simulink model "Four_DoF_02_2023b"  (R2024a)
settings: Solver=ode1be  StartTime=0.0  StopTime=inf  FixedStep=0.001  RelTol=1e-3
undefined symbols (not defined in the file or in its folder): X, Y, Z
libraries: sm_lib x127, nesl_utility x70, robotcorelib x6
(part 3 of 3)

== system Four_DoF_02_2023b/Gravity Corn(FF controller)1 ==
  note: mgLsin(zeta)
  q : Inport
  Sin : Trigonometry
  mg : Gain  Gain=1*9.80665*1
  Out1 : Outport
  wires:
  Sin/1 -> mg/1
  q/1 -> Sin/1
  mg/1 -> Out1/1

== system Four_DoF_02_2023b/Gravity Corn(FF controller)2 ==
  note: mgLsin(zeta)
  q : Inport
  Sin : Trigonometry
  mg : Gain  Gain=1*9.80665*1
  Out1 : Outport
  wires:
  Sin/1 -> mg/1
  q/1 -> Sin/1
  mg/1 -> Out1/1

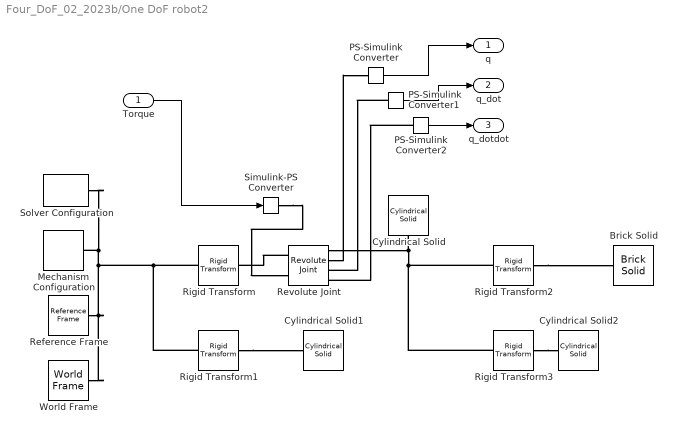
== system Four_DoF_02_2023b/One DoF robot2 ==
  Torque : Inport
  Brick Solid : sm_lib/Body Elements/Brick Solid  BrickDimensions=[0.1 0.1 0.1]  BrickDimensionsUnits=m  ExportEntireGeometry=off  InertiaType=PointMass  BasedOnType=Density  Density=1000  DensityUnits=kg/m^3  Mass=1  MassUnits=kg  CenterOfMass=[0 0 0]  CenterOfMassUnits=m  MomentsOfInertia=[1 1 1]  MomentsOfInertiaUnits=kg*m^2  ProductsOfInertia=[0 0 0]  ProductsOfInertiaUnits=kg*m^2  GraphicType=FromGeometry  MarkerShape=Sphere  MarkerSize=10  GraphicVisPropType=SimpleVisualProperties  GraphicDiffuseColor=[0.5 0.5 0.5]  GraphicOpacity=1.0  GraphicSpecularColor=[0.5 0.5 0.5 1.0]  GraphicAmbientColor=[0.15 0.15 0.15 1.0]  GraphicEmissiveColor=[0.0 0.0 0.0 1.0]  GraphicShininess=75  DoExposeReferenceFrame=on  SerializedFrames=<Frames/>
  Cylindrical Solid : sm_lib/Body Elements/Cylindrical Solid  CylinderRadius=0.05  CylinderRadiusUnits=m  CylinderLength=0.1  CylinderLengthUnits=m  ExportEntireGeometry=off  InertiaType=PointMass  BasedOnType=Density  Density=1000  DensityUnits=kg/m^3  Mass=0.0001  MassUnits=kg  CenterOfMass=[0 0 0]  CenterOfMassUnits=m  MomentsOfInertia=[1 1 1]  MomentsOfInertiaUnits=kg*m^2  ProductsOfInertia=[0 0 0]  ProductsOfInertiaUnits=kg*m^2  GraphicType=FromGeometry  MarkerShape=Sphere  MarkerSize=10  GraphicVisPropType=SimpleVisualProperties  GraphicDiffuseColor=[1.0 0.0 0.2]  GraphicOpacity=1.0  GraphicSpecularColor=[0.5 0.5 0.5 1.0]  GraphicAmbientColor=[0.15 0.15 0.15 1.0]  GraphicEmissiveColor=[0.0 0.0 0.0 1.0]  GraphicShininess=75  DoExposeReferenceFrame=on  SerializedFrames=<Frames/>
  Cylindrical Solid1 : sm_lib/Body Elements/Cylindrical Solid  CylinderRadius=0.02  CylinderRadiusUnits=m  CylinderLength=0.5  CylinderLengthUnits=m  ExportEntireGeometry=off  InertiaType=PointMass  BasedOnType=Density  Density=1000  DensityUnits=kg/m^3  Mass=0.001  MassUnits=kg  CenterOfMass=[0 0 0]  CenterOfMassUnits=m  MomentsOfInertia=[1 1 1]  MomentsOfInertiaUnits=kg*m^2  ProductsOfInertia=[0 0 0]  ProductsOfInertiaUnits=kg*m^2  GraphicType=FromGeometry  MarkerShape=Sphere  MarkerSize=10  GraphicVisPropType=SimpleVisualProperties  GraphicDiffuseColor=[1.0 0.6 0.2]  GraphicOpacity=1.0  GraphicSpecularColor=[0.5 0.5 0.5 1.0]  GraphicAmbientColor=[0.15 0.15 0.15 1.0]  GraphicEmissiveColor=[0.0 0.0 0.0 1.0]  GraphicShininess=75  DoExposeReferenceFrame=on  SerializedFrames=<Frames/>
  Cylindrical Solid2 : sm_lib/Body Elements/Cylindrical Solid  CylinderRadius=0.02  CylinderRadiusUnits=m  CylinderLength=1  CylinderLengthUnits=m  ExportEntireGeometry=off  InertiaType=PointMass  BasedOnType=Density  Density=1000  DensityUnits=kg/m^3  Mass=0.001  MassUnits=kg  CenterOfMass=[0 0 0]  CenterOfMassUnits=m  MomentsOfInertia=[1 1 1]  MomentsOfInertiaUnits=kg*m^2  ProductsOfInertia=[0 0 0]  ProductsOfInertiaUnits=kg*m^2  GraphicType=FromGeometry  MarkerShape=Sphere  MarkerSize=10  GraphicVisPropType=SimpleVisualProperties  GraphicDiffuseColor=[1.0 0.6 0.2]  GraphicOpacity=1.0  GraphicSpecularColor=[0.5 0.5 0.5 1.0]  GraphicAmbientColor=[0.15 0.15 0.15 1.0]  GraphicEmissiveColor=[0.0 0.0 0.0 1.0]  GraphicShininess=75  DoExposeReferenceFrame=on  SerializedFrames=<Frames/>
  Mechanism Configuration : sm_lib/Utilities/Mechanism Configuration  UniformGravity=Constant  GravityVector=[0 0 -9.80665]  GravityVectorUnits=m/s^2  LinearizationDelta=0.001  JointModeTransitionNonlinearIterations=2
  PS-Simulink Converter : nesl_utility/PS-Simulink Converter  PhysicalDomain=network_engine_domain  SubClassName=ps_output  LeftPortType=input  RightPortType=output  PseudoPeriodic=off  Frequencies=[]  VectorFormat=inherit  Unit=inherit  AffineConversion=off
  PS-Simulink Converter1 : nesl_utility/PS-Simulink Converter  PhysicalDomain=network_engine_domain  SubClassName=ps_output  LeftPortType=input  RightPortType=output  PseudoPeriodic=off  Frequencies=[]  VectorFormat=inherit  Unit=inherit  AffineConversion=off
  PS-Simulink Converter2 : nesl_utility/PS-Simulink Converter  PhysicalDomain=network_engine_domain  SubClassName=ps_output  LeftPortType=input  RightPortType=output  PseudoPeriodic=off  Frequencies=[]  VectorFormat=inherit  Unit=inherit  AffineConversion=off
  Reference Frame : sm_lib/Frames and Transforms/Reference Frame
  Revolute Joint : sm_lib/Joints/Revolute Joint  JointMode=Normal  CompositeWrenchDir=FollowerOnBase  CompositeWrenchFrame=BaseFrame  SenseConstraintForce=off  SenseConstraintTorque=off  SenseTotalForce=off  SenseTotalTorque=off  PositionTargetSpecify=on  PositionTargetPriority=High  PositionTargetValue=45  PositionTargetValueUnits=deg  VelocityTargetSpecify=off  VelocityTargetPriority=High  VelocityTargetValue=0  VelocityTargetValueUnits=deg/s  EquilibriumPosition=0  EquilibriumPositionUnits=deg  SpringStiffness=0  SpringStiffnessUnits=N*m/deg  DampingCoefficient=0.01  DampingCoefficientUnits=N*m/(deg/s)  LowerLimitSpecify=off  LowerLimitBound=-90  LowerLimitBoundUnits=deg  LowerLimitStiffness=1e4  LowerLimitStiffnessUnits=N*m/deg  LowerLimitDamping=10  LowerLimitDampingUnits=N*m/(deg/s)  LowerLimitTransitionRegionWidth=0.1  LowerLimitTransitionRegionWidthUnits=deg  UpperLimitSpecify=off  UpperLimitBound=90  UpperLimitBoundUnits=deg  UpperLimitStiffness=1e4  UpperLimitStiffnessUnits=N*m/deg  UpperLimitDamping=10  UpperLimitDampingUnits=N*m/(deg/s)  UpperLimitTransitionRegionWidth=0.1  UpperLimitTransitionRegionWidthUnits=deg  TorqueActuationMode=InputTorque  MotionActuationMode=ComputedMotion  SensePosition=on  SenseVelocity=on  SenseAcceleration=on  SenseTorqueForce=off  SenseLowerLimitTorqueForce=off  SenseUpperLimitTorqueForce=off
  Rigid Transform : sm_lib/Frames and Transforms/Rigid Transform  RotationMethod=StandardAxis  FollAlignAxisA=+X  BaseAlignAxisA=+Y  FollAlignAxisB=+Y  BaseAlignAxisB=+Z  RotationStandardAxis=+Y  RotationAngle=90  RotationAngleUnits=deg  RotationArbitraryAxis=[0 0 1]  RotationSequenceAxes=FollowerAxes  RotationSequence=XYX  RotationSequenceAngles=[0 0 0]  RotationSequenceAnglesUnits=deg  RotationMatrix=[1 0 0; 0 1 0; 0 0 1]  Quaternion=[1 0 0 0]  TranslationMethod=Cartesian  TranslationCartesianOffset=[0 0 0.5]  TranslationCartesianOffsetUnits=m  TranslationStandardAxis=+Z  TranslationStandardOffset=0  TranslationStandardOffsetUnits=m  TranslationROffset=0  TranslationROffsetUnits=m  TranslationThetaOffset=0  TranslationThetaOffsetUnits=deg  TranslationZOffset=0  TranslationZOffsetUnits=m
  Rigid Transform1 : sm_lib/Frames and Transforms/Rigid Transform  RotationMethod=None  FollAlignAxisA=+X  BaseAlignAxisA=+Y  FollAlignAxisB=+Y  BaseAlignAxisB=+Z  RotationStandardAxis=+Y  RotationAngle=90  RotationAngleUnits=deg  RotationArbitraryAxis=[0 0 1]  RotationSequenceAxes=FollowerAxes  RotationSequence=XYX  RotationSequenceAngles=[0 0 0]  RotationSequenceAnglesUnits=deg  RotationMatrix=[1 0 0; 0 1 0; 0 0 1]  Quaternion=[1 0 0 0]  TranslationMethod=Cartesian  TranslationCartesianOffset=[0 0 0.25]  TranslationCartesianOffsetUnits=m  TranslationStandardAxis=+Z  TranslationStandardOffset=0  TranslationStandardOffsetUnits=m  TranslationROffset=0  TranslationROffsetUnits=m  TranslationThetaOffset=0  TranslationThetaOffsetUnits=deg  TranslationZOffset=0  TranslationZOffsetUnits=m
  Rigid Transform2 : sm_lib/Frames and Transforms/Rigid Transform  RotationMethod=None  FollAlignAxisA=+X  BaseAlignAxisA=+Y  FollAlignAxisB=+Y  BaseAlignAxisB=+Z  RotationStandardAxis=+Z  RotationAngle=0.0  RotationAngleUnits=deg  RotationArbitraryAxis=[0 0 1]  RotationSequenceAxes=FollowerAxes  RotationSequence=XYX  RotationSequenceAngles=[0 0 0]  RotationSequenceAnglesUnits=deg  RotationMatrix=[1 0 0; 0 1 0; 0 0 1]  Quaternion=[1 0 0 0]  TranslationMethod=Cartesian  TranslationCartesianOffset=[1 0 0]  TranslationCartesianOffsetUnits=m  TranslationStandardAxis=+Z  TranslationStandardOffset=0  TranslationStandardOffsetUnits=m  TranslationROffset=0  TranslationROffsetUnits=m  TranslationThetaOffset=0  TranslationThetaOffsetUnits=deg  TranslationZOffset=0  TranslationZOffsetUnits=m
  Rigid Transform3 : sm_lib/Frames and Transforms/Rigid Transform  RotationMethod=StandardAxis  FollAlignAxisA=+X  BaseAlignAxisA=+Y  FollAlignAxisB=+Y  BaseAlignAxisB=+Z  RotationStandardAxis=+Y  RotationAngle=90  RotationAngleUnits=deg  RotationArbitraryAxis=[0 0 1]  RotationSequenceAxes=FollowerAxes  RotationSequence=XYX  RotationSequenceAngles=[0 0 0]  RotationSequenceAnglesUnits=deg  RotationMatrix=[1 0 0; 0 1 0; 0 0 1]  Quaternion=[1 0 0 0]  TranslationMethod=Cartesian  TranslationCartesianOffset=[0.5 0 0]  TranslationCartesianOffsetUnits=m  TranslationStandardAxis=+Z  TranslationStandardOffset=0  TranslationStandardOffsetUnits=m  TranslationROffset=0  TranslationROffsetUnits=m  TranslationThetaOffset=0  TranslationThetaOffsetUnits=deg  TranslationZOffset=0  TranslationZOffsetUnits=m
  Simulink-PS Converter : nesl_utility/Simulink-PS Converter  PhysicalDomain=network_engine_domain  SubClassName=ps_input  LeftPortType=input  RightPortType=output  PseudoPeriodic=off  Frequencies=[]  NoiseDistribution=none  NoiseParameters=[]  Unit=1  AffineConversion=off  FilteringAndDerivatives=provide  SimscapeFilterOrder=1  InputFilterTimeConstant=0.001  UdotUserProvided=0
  Solver Configuration : nesl_utility/Solver Configuration  PhysicalDomain=network_engine_domain  SubClassName=solver  LeftPortType=input  RightPortType=generic  Tones=[]  Harmonics=[]  SimulateNoise=off  Profile=off  UseLocalSampling=off  EnableSwitchedLinearOptims=on  FrequencyDomain=off  UseCCode=off  RelTol=0.001  AbsTol=0.001  MinStep=1e-09  ToWorkspace=off  RevertToSquareIcSolve=off  NumHomotopyIterations=100  PhasorMode=off  PhasorModeNumHarmonics=1  ConsistencySolver=NEWTON_XTOL_AFTER_FTOL  IndexReductionMethod=DerivativeReplacement  DoDC=off  ResidualTolerance=1e-09  ConsistencyTolSource=GLOBAL  ConsistencyAbsTol=0.001  ConsistencyRelTol=0.001  ConsistencyTolFactor=0.001  UseLocalSolver=off  LocalSolverChoice=NE_BACKWARD_EULER_ADVANCER  ResolveIndetEquations=on  FunctionEvalNumThread=1  LocalSolverSampleTime=0.001  DoFixedCost=off  MaxNonlinIter=3  MaxModeIter=2  ComputeImpulses=off  ImpulseIterations=2  LinearAlgebra=auto  LinearAlgebraNumThread=0  EquationFormulation=NE_TIME_EF  DelaysMemoryBudget=1024  AutomaticFiltering=on  FilteringTimeConstant=0.001  PartitionStorageMethod=AS_NEEDED  PartitionMemoryBudget=1024  PartitionMethod=ROBUST  MultibodyUseLocalSolver=off  MultibodyLocalSolverChoice=ODE1  MultibodyLocalSolverSampleTime=0.001
  World Frame : sm_lib/Frames and Transforms/World Frame
  q : Outport
  q_dot : Outport  Port=2
  q_dotdot : Outport  Port=3
  wires:
  Torque/1 -> Simulink-PS Converter/1
  PS-Simulink Converter/1 -> q/1
  PS-Simulink Converter2/1 -> q_dotdot/1
  PS-Simulink Converter1/1 -> q_dot/1
  connections:
  Solver Configuration/RConn1 -- Rigid Transform1/LConn1 -- Rigid Transform/LConn1 -- World Frame/RConn1 -- Reference Frame/RConn1 -- Mechanism Configuration/RConn1
  Revolute Joint/RConn1 -- Rigid Transform3/LConn1 -- Rigid Transform2/LConn1 -- Cylindrical Solid/RConn1
  Revolute Joint/LConn1 -- Rigid Transform/RConn1
  Rigid Transform3/RConn1 -- Cylindrical Solid2/RConn1
  Rigid Transform1/RConn1 -- Cylindrical Solid1/RConn1
  PS-Simulink Converter2/LConn1 -- Revolute Joint/RConn4
  Revolute Joint/RConn2 -- PS-Simulink Converter/LConn1
  Rigid Transform2/RConn1 -- Brick Solid/RConn1
  Simulink-PS Converter/RConn1 -- Revolute Joint/LConn2
  PS-Simulink Converter1/LConn1 -- Revolute Joint/RConn3

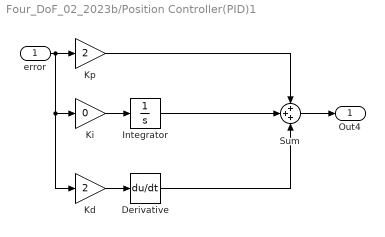
== system Four_DoF_02_2023b/Position Controller(PID)1 ==
  error : Inport
  Derivative : Derivative
  Integrator : Integrator
  Kd : Gain  Gain=2
  Ki : Gain  Gain=0
  Kp : Gain  Gain=2
  Sum : Sum  Inputs=+++
  Out4 : Outport
  wires:
  Derivative/1 -> Sum/3
  Ki/1 -> Integrator/1
  Integrator/1 -> Sum/2
  Kd/1 -> Derivative/1
  Kp/1 -> Sum/1
  error/1 -> Kd/1, Ki/1, Kp/1
  Sum/1 -> Out4/1

== system Four_DoF_02_2023b/Position Controller(PID)2 ==
  error : Inport
  Derivative : Derivative
  Integrator : Integrator
  Kd : Gain  Gain=2
  Ki : Gain  Gain=0
  Kp : Gain  Gain=2
  Sum : Sum  Inputs=+++
  Out4 : Outport
  wires:
  Derivative/1 -> Sum/3
  Ki/1 -> Integrator/1
  Integrator/1 -> Sum/2
  Kd/1 -> Derivative/1
  Kp/1 -> Sum/1
  error/1 -> Kd/1, Ki/1, Kp/1
  Sum/1 -> Out4/1

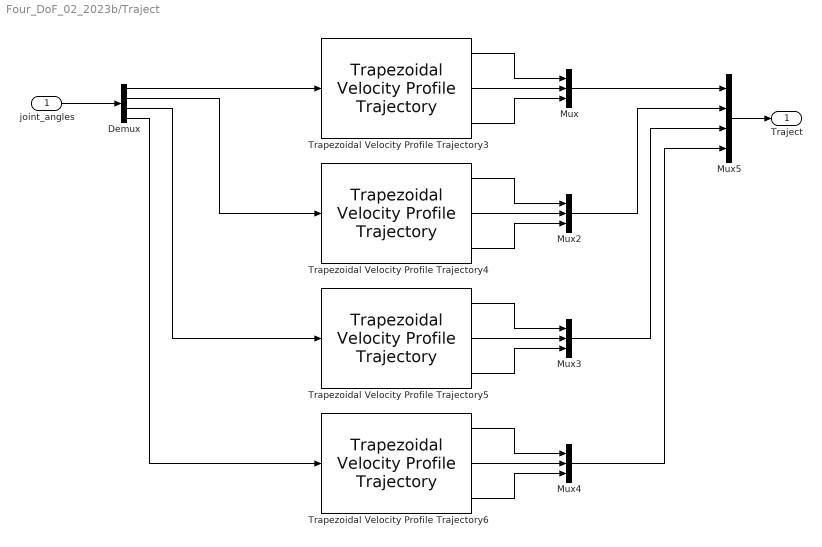
== system Four_DoF_02_2023b/Traject ==
  joint_angles : Inport
  Demux : Demux
  Mux{,2..4} (4 alike) : Mux  Inputs=3
  Mux5 : Mux
  Trapezoidal Velocity Profile Trajectory3 : robotcorelib/Trapezoidal Velocity Profile Trajectory  WaypointSource=Internal  Waypoints=[ 0, 0, 0]  NumParams=0  Parameter1=Peak Velocity  Parameter2=End Time  ParameterSource=Internal  PeakVelocity=[ 2; 2 ]  Acceleration=[ 1; 2 ]  EndTime=[ 1; 1 ]  AccelTime=[ 1; 2 ]  SimulateUsing=Interpreted execution
  Trapezoidal Velocity Profile Trajectory4 : robotcorelib/Trapezoidal Velocity Profile Trajectory  WaypointSource=Internal  Waypoints=[ 0, 0, 0]  NumParams=0  Parameter1=Peak Velocity  Parameter2=End Time  ParameterSource=Internal  PeakVelocity=[ 2; 2 ]  Acceleration=[ 1; 2 ]  EndTime=[ 1; 1 ]  AccelTime=[ 1; 2 ]  SimulateUsing=Interpreted execution
  Trapezoidal Velocity Profile Trajectory5 : robotcorelib/Trapezoidal Velocity Profile Trajectory  WaypointSource=Internal  Waypoints=[ 0, 1, 5]  NumParams=0  Parameter1=Peak Velocity  Parameter2=End Time  ParameterSource=Internal  PeakVelocity=[ 2; 2 ]  Acceleration=[ 1; 2 ]  EndTime=[ 1; 1 ]  AccelTime=[ 1; 2 ]  SimulateUsing=Interpreted execution
  Trapezoidal Velocity Profile Trajectory6 : robotcorelib/Trapezoidal Velocity Profile Trajectory  WaypointSource=Internal  Waypoints=[ 0, 1, 3]  NumParams=0  Parameter1=Peak Velocity  Parameter2=End Time  ParameterSource=Internal  PeakVelocity=[ 2; 2 ]  Acceleration=[ 1; 2 ]  EndTime=[ 1; 1 ]  AccelTime=[ 1; 2 ]  SimulateUsing=Interpreted execution
  Traject : Outport
  wires:
  Trapezoidal Velocity Profile Trajectory5/2 -> Mux3/2
  Mux4/1 -> Mux5/4
  Mux3/1 -> Mux5/3
  Trapezoidal Velocity Profile Trajectory3/2 -> Mux/2
  Trapezoidal Velocity Profile Trajectory6/1 -> Mux4/1
  Mux2/1 -> Mux5/2
  Trapezoidal Velocity Profile Trajectory6/2 -> Mux4/2
  Trapezoidal Velocity Profile Trajectory3/3 -> Mux/3
  Trapezoidal Velocity Profile Trajectory6/3 -> Mux4/3
  Trapezoidal Velocity Profile Trajectory5/3 -> Mux3/3
  Trapezoidal Velocity Profile Trajectory3/1 -> Mux/1
  Mux/1 -> Mux5/1
  Trapezoidal Velocity Profile Trajectory4/3 -> Mux2/3
  Trapezoidal Velocity Profile Trajectory4/1 -> Mux2/1
  Trapezoidal Velocity Profile Trajectory4/2 -> Mux2/2
  Trapezoidal Velocity Profile Trajectory5/1 -> Mux3/1
  Mux5/1 -> Traject/1
  joint_angles/1 -> Demux/1
  Demux/1 -> Trapezoidal Velocity Profile Trajectory3/1
  Demux/2 -> Trapezoidal Velocity Profile Trajectory4/1
  Demux/3 -> Trapezoidal Velocity Profile Trajectory5/1
  Demux/4 -> Trapezoidal Velocity Profile Trajectory6/1

== system Four_DoF_02_2023b/Velocity Controller(PID)1 ==
  error : Inport
  Derivative : Derivative
  Integrator : Integrator
  Kd : Gain  Gain=0
  Ki : Gain  Gain=0
  Kp : Gain  Gain=4
  Sum : Sum  Inputs=+++
  Out4 : Outport
  wires:
  Derivative/1 -> Sum/3
  Ki/1 -> Integrator/1
  Integrator/1 -> Sum/2
  Kd/1 -> Derivative/1
  Kp/1 -> Sum/1
  error/1 -> Kd/1, Ki/1, Kp/1
  Sum/1 -> Out4/1

== system Four_DoF_02_2023b/Velocity Controller(PID)2 ==
  error : Inport
  Derivative : Derivative
  Integrator : Integrator
  Kd : Gain  Gain=0
  Ki : Gain  Gain=0
  Kp : Gain
  Sum : Sum  Inputs=+++
  Torque 2 : Outport
  wires:
  Derivative/1 -> Sum/3
  Ki/1 -> Integrator/1
  Integrator/1 -> Sum/2
  Kd/1 -> Derivative/1
  Kp/1 -> Sum/1
  error/1 -> Kd/1, Ki/1, Kp/1
  Sum/1 -> Torque 2/1

== system Four_DoF_02_2023b/Velocity Controller(PID)3 ==
  error : Inport
  Derivative : Derivative
  Integrator : Integrator
  Kd : Gain  Gain=0
  Ki : Gain  Gain=0
  Kp : Gain  Gain=4
  Sum : Sum  Inputs=+++
  Out4 : Outport
  wires:
  Derivative/1 -> Sum/3
  Ki/1 -> Integrator/1
  Integrator/1 -> Sum/2
  Kd/1 -> Derivative/1
  Kp/1 -> Sum/1
  error/1 -> Kd/1, Ki/1, Kp/1
  Sum/1 -> Out4/1

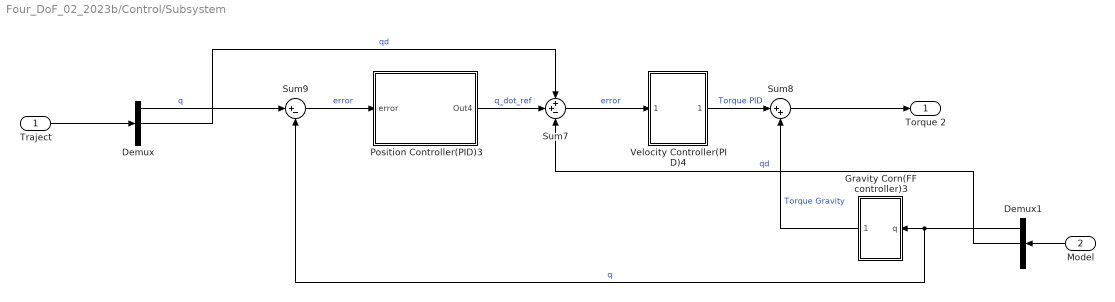
== system Four_DoF_02_2023b/Control/Subsystem ==
  Traject : Inport
  Model : Inport  Port=2
  Demux : Demux  Outputs=3
  Demux1 : Demux  Outputs=3
  Gravity Corn(FF controller)3 : Subsystem
  Position Controller(PID)3 : Subsystem
  Sum7 : Sum  Inputs=++-
  Sum8 : Sum  Inputs=|++
  Sum9 : Sum  Inputs=|+-
  Velocity Controller(PID)4 : Subsystem
  Torque 2 : Outport
  wires:
  Position Controller(PID)3/1(Out4) -> Sum7/2  "q_dot_ref"
  Gravity Corn(FF controller)3/1(Out1) -> Sum8/2  "Torque Gravity"
  Traject/1 -> Demux/1
  Velocity Controller(PID)4/1(Out4) -> Sum8/1  "Torque PID"
  Sum7/1 -> Velocity Controller(PID)4/1(error)  "error"
  Sum9/1 -> Position Controller(PID)3/1(error)  "error"
  Sum8/1 -> Torque 2/1
  Demux/1 -> Sum9/1  "q"
  Demux/2 -> Sum7/1  "qd"
  Model/1 -> Demux1/1
  Demux1/1 -> Sum9/2, Gravity Corn(FF controller)3/1(q)  "q"
  Demux1/2 -> Sum7/3  "qd"

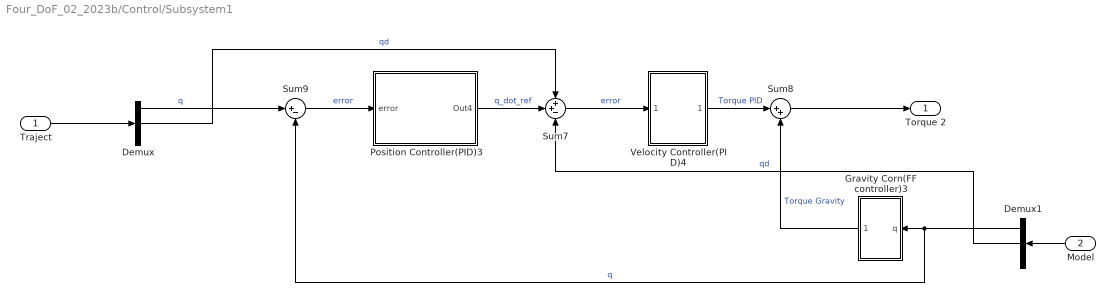
== system Four_DoF_02_2023b/Control/Subsystem1 ==
  Traject : Inport
  Model : Inport  Port=2
  Demux : Demux  Outputs=3
  Demux1 : Demux  Outputs=3
  Gravity Corn(FF controller)3 : Subsystem
  Position Controller(PID)3 : Subsystem
  Sum7 : Sum  Inputs=++-
  Sum8 : Sum  Inputs=|++
  Sum9 : Sum  Inputs=|+-
  Velocity Controller(PID)4 : Subsystem
  Torque 2 : Outport
  wires:
  Position Controller(PID)3/1(Out4) -> Sum7/2  "q_dot_ref"
  Gravity Corn(FF controller)3/1(Out1) -> Sum8/2  "Torque Gravity"
  Traject/1 -> Demux/1
  Velocity Controller(PID)4/1(Out4) -> Sum8/1  "Torque PID"
  Sum7/1 -> Velocity Controller(PID)4/1(error)  "error"
  Sum9/1 -> Position Controller(PID)3/1(error)  "error"
  Sum8/1 -> Torque 2/1
  Demux/1 -> Sum9/1  "q"
  Demux/2 -> Sum7/1  "qd"
  Model/1 -> Demux1/1
  Demux1/1 -> Sum9/2, Gravity Corn(FF controller)3/1(q)  "q"
  Demux1/2 -> Sum7/3  "qd"

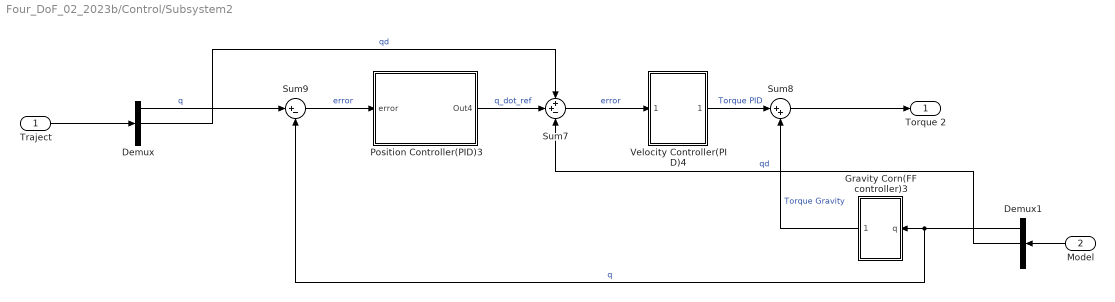
== system Four_DoF_02_2023b/Control/Subsystem2 ==
  Traject : Inport
  Model : Inport  Port=2
  Demux : Demux  Outputs=3
  Demux1 : Demux  Outputs=3
  Gravity Corn(FF controller)3 : Subsystem
  Position Controller(PID)3 : Subsystem
  Sum7 : Sum  Inputs=++-
  Sum8 : Sum  Inputs=|++
  Sum9 : Sum  Inputs=|+-
  Velocity Controller(PID)4 : Subsystem
  Torque 2 : Outport
  wires:
  Position Controller(PID)3/1(Out4) -> Sum7/2  "q_dot_ref"
  Gravity Corn(FF controller)3/1(Out1) -> Sum8/2  "Torque Gravity"
  Traject/1 -> Demux/1
  Velocity Controller(PID)4/1(Out4) -> Sum8/1  "Torque PID"
  Sum7/1 -> Velocity Controller(PID)4/1(error)  "error"
  Sum9/1 -> Position Controller(PID)3/1(error)  "error"
  Sum8/1 -> Torque 2/1
  Demux/1 -> Sum9/1  "q"
  Demux/2 -> Sum7/1  "qd"
  Model/1 -> Demux1/1
  Demux1/1 -> Sum9/2, Gravity Corn(FF controller)3/1(q)  "q"
  Demux1/2 -> Sum7/3  "qd"

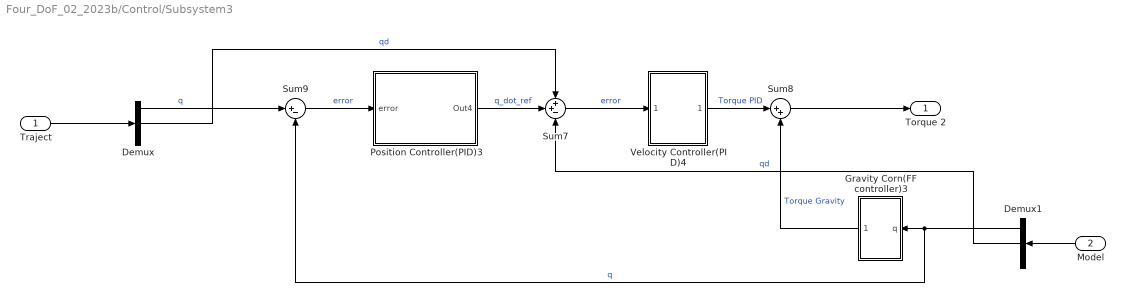
== system Four_DoF_02_2023b/Control/Subsystem3 ==
  Traject : Inport
  Model : Inport  Port=2
  Demux : Demux  Outputs=3
  Demux1 : Demux  Outputs=3
  Gravity Corn(FF controller)3 : Subsystem
  Position Controller(PID)3 : Subsystem
  Sum7 : Sum  Inputs=++-
  Sum8 : Sum  Inputs=|++
  Sum9 : Sum  Inputs=|+-
  Velocity Controller(PID)4 : Subsystem
  Torque 2 : Outport
  wires:
  Position Controller(PID)3/1(Out4) -> Sum7/2  "q_dot_ref"
  Gravity Corn(FF controller)3/1(Out1) -> Sum8/2  "Torque Gravity"
  Traject/1 -> Demux/1
  Velocity Controller(PID)4/1(Out4) -> Sum8/1  "Torque PID"
  Sum7/1 -> Velocity Controller(PID)4/1(error)  "error"
  Sum9/1 -> Position Controller(PID)3/1(error)  "error"
  Sum8/1 -> Torque 2/1
  Demux/1 -> Sum9/1  "q"
  Demux/2 -> Sum7/1  "qd"
  Model/1 -> Demux1/1
  Demux1/1 -> Sum9/2, Gravity Corn(FF controller)3/1(q)  "q"
  Demux1/2 -> Sum7/3  "qd"

== system Four_DoF_02_2023b/Control/Subsystem/Gravity Corn(FF controller)3 ==
  note: mgLsin(zeta)
  q : Inport
  Sin : Trigonometry
  mg : Gain  Gain=1*9.80665*1
  Out1 : Outport
  wires:
  Sin/1 -> mg/1
  q/1 -> Sin/1
  mg/1 -> Out1/1

== system Four_DoF_02_2023b/Control/Subsystem/Position Controller(PID)3 ==
  error : Inport
  Derivative : Derivative
  Integrator : Integrator
  Kd : Gain  Gain=2
  Ki : Gain  Gain=0
  Kp : Gain  Gain=2
  Sum : Sum  Inputs=+++
  Out4 : Outport
  wires:
  Derivative/1 -> Sum/3
  Ki/1 -> Integrator/1
  Integrator/1 -> Sum/2
  Kd/1 -> Derivative/1
  Kp/1 -> Sum/1
  error/1 -> Kd/1, Ki/1, Kp/1
  Sum/1 -> Out4/1

== system Four_DoF_02_2023b/Control/Subsystem/Velocity Controller(PID)4 ==
  error : Inport
  Derivative : Derivative
  Integrator : Integrator
  Kd : Gain  Gain=0
  Ki : Gain  Gain=0
  Kp : Gain  Gain=4
  Sum : Sum  Inputs=+++
  Out4 : Outport
  wires:
  Derivative/1 -> Sum/3
  Ki/1 -> Integrator/1
  Integrator/1 -> Sum/2
  Kd/1 -> Derivative/1
  Kp/1 -> Sum/1
  error/1 -> Kd/1, Ki/1, Kp/1
  Sum/1 -> Out4/1

== system Four_DoF_02_2023b/Control/Subsystem1/Gravity Corn(FF controller)3 ==
  note: mgLsin(zeta)
  q : Inport
  Sin : Trigonometry
  mg : Gain  Gain=1*9.80665*1
  Out1 : Outport
  wires:
  Sin/1 -> mg/1
  q/1 -> Sin/1
  mg/1 -> Out1/1

== system Four_DoF_02_2023b/Control/Subsystem1/Position Controller(PID)3 ==
  error : Inport
  Derivative : Derivative
  Integrator : Integrator
  Kd : Gain  Gain=2
  Ki : Gain  Gain=0
  Kp : Gain  Gain=2
  Sum : Sum  Inputs=+++
  Out4 : Outport
  wires:
  Derivative/1 -> Sum/3
  Ki/1 -> Integrator/1
  Integrator/1 -> Sum/2
  Kd/1 -> Derivative/1
  Kp/1 -> Sum/1
  error/1 -> Kd/1, Ki/1, Kp/1
  Sum/1 -> Out4/1

== system Four_DoF_02_2023b/Control/Subsystem1/Velocity Controller(PID)4 ==
  error : Inport
  Derivative : Derivative
  Integrator : Integrator
  Kd : Gain  Gain=0
  Ki : Gain  Gain=0
  Kp : Gain  Gain=4
  Sum : Sum  Inputs=+++
  Out4 : Outport
  wires:
  Derivative/1 -> Sum/3
  Ki/1 -> Integrator/1
  Integrator/1 -> Sum/2
  Kd/1 -> Derivative/1
  Kp/1 -> Sum/1
  error/1 -> Kd/1, Ki/1, Kp/1
  Sum/1 -> Out4/1

== system Four_DoF_02_2023b/Control/Subsystem2/Gravity Corn(FF controller)3 ==
  note: mgLsin(zeta)
  q : Inport
  Sin : Trigonometry
  mg : Gain  Gain=1*9.80665*1
  Out1 : Outport
  wires:
  Sin/1 -> mg/1
  q/1 -> Sin/1
  mg/1 -> Out1/1

== system Four_DoF_02_2023b/Control/Subsystem2/Position Controller(PID)3 ==
  error : Inport
  Derivative : Derivative
  Integrator : Integrator
  Kd : Gain  Gain=2
  Ki : Gain  Gain=0
  Kp : Gain  Gain=2
  Sum : Sum  Inputs=+++
  Out4 : Outport
  wires:
  Derivative/1 -> Sum/3
  Ki/1 -> Integrator/1
  Integrator/1 -> Sum/2
  Kd/1 -> Derivative/1
  Kp/1 -> Sum/1
  error/1 -> Kd/1, Ki/1, Kp/1
  Sum/1 -> Out4/1

== system Four_DoF_02_2023b/Control/Subsystem2/Velocity Controller(PID)4 ==
  error : Inport
  Derivative : Derivative
  Integrator : Integrator
  Kd : Gain  Gain=0
  Ki : Gain  Gain=0
  Kp : Gain  Gain=4
  Sum : Sum  Inputs=+++
  Out4 : Outport
  wires:
  Derivative/1 -> Sum/3
  Ki/1 -> Integrator/1
  Integrator/1 -> Sum/2
  Kd/1 -> Derivative/1
  Kp/1 -> Sum/1
  error/1 -> Kd/1, Ki/1, Kp/1
  Sum/1 -> Out4/1

== system Four_DoF_02_2023b/Control/Subsystem3/Gravity Corn(FF controller)3 ==
  note: mgLsin(zeta)
  q : Inport
  Sin : Trigonometry
  mg : Gain  Gain=1*9.80665*1
  Out1 : Outport
  wires:
  Sin/1 -> mg/1
  q/1 -> Sin/1
  mg/1 -> Out1/1

== system Four_DoF_02_2023b/Control/Subsystem3/Position Controller(PID)3 ==
  error : Inport
  Derivative : Derivative
  Integrator : Integrator
  Kd : Gain  Gain=2
  Ki : Gain  Gain=0
  Kp : Gain  Gain=2
  Sum : Sum  Inputs=+++
  Out4 : Outport
  wires:
  Derivative/1 -> Sum/3
  Ki/1 -> Integrator/1
  Integrator/1 -> Sum/2
  Kd/1 -> Derivative/1
  Kp/1 -> Sum/1
  error/1 -> Kd/1, Ki/1, Kp/1
  Sum/1 -> Out4/1

== system Four_DoF_02_2023b/Control/Subsystem3/Velocity Controller(PID)4 ==
  error : Inport
  Derivative : Derivative
  Integrator : Integrator
  Kd : Gain  Gain=0
  Ki : Gain  Gain=0
  Kp : Gain  Gain=4
  Sum : Sum  Inputs=+++
  Out4 : Outport
  wires:
  Derivative/1 -> Sum/3
  Ki/1 -> Integrator/1
  Integrator/1 -> Sum/2
  Kd/1 -> Derivative/1
  Kp/1 -> Sum/1
  error/1 -> Kd/1, Ki/1, Kp/1
  Sum/1 -> Out4/1

== matlab function Four_DoF_02_2023b/MATLAB Function1 ==
  data: joint_angles input; x output; y output; z output; phi output
function [x, y, z, phi] = FK_Simulink(joint_angles)
    % FK_Simulink: Calculates the position and orientation of the end effector for a 4-DOF manipulator

    % Lengths of the links
    L1 = 0.25; % Link 1
    L2 = 1; % Link 2
    L3 = 1.5; % Link 3
    L4 = 0.75; % Link 4 (End Effector)

    % Extract joint angles
    q1 = joint_angles(1); % Joint 1 (base rotation)
    q2 = joint_angles(2); % Joint 2 (shoulder rotation)
    q3 = joint_angles(3); % Joint 3 (elbow rotation)
    q4 = joint_angles(4); % Joint 4 (end effector orientation)

    % Transformation Matrices
    % Transform from base frame to end effector
    % Transformation for Joint 1 (Rotation around the base)
    T1 = [cos(q1), -sin(q1), 0, 0;
          sin(q1), cos(q1), 0, 0;
          0, 0, 1, L1;
          0, 0, 0, 1];

    % Transformation for Joint 2 (shoulder)
    T2 = [cos(q2), -sin(q2), 0, 0;
           0, 0, -1, 0;
          sin(q2), cos(q2), 0, 0;
          0, 0, 0, 1];

    % Transformation for Joint 3 (elbow)
    T3 = [cos(q3), -sin(q3), 0, L2;
          sin(q3), cos(q3), 0, 0;
          0, 0, 1, 0;
          0, 0, 0, 1];

    % Transformation for Joint 4 (end effector orientation)
    T4 = [cos(q4), -sin(q4), 0, L3;
          sin(q4), cos(q4), 0, 0;
          0, 0, 1, 0;
          0, 0, 0, 1];

    T5 = [1, 0, 0, L4;
      0, 1, 0, 0;
      0, 0, 1, 0;
      0, 0, 0, 1];

    % Final transformation from the base to end effector
    T = T1 * T2 * T3 * T4 * T5;

    % Extract position from the final transformation matrix
    x = T(1, 4); % x-position of the end effector
    y = T(2, 4); % y-position of the end effector
    z = T(3, 4); % z-position of the end effector

    % Extract orientation (phi) from the transformation matrix
    phi = atan2(T(2, 1), T(1, 1)); % Rotation around the z-axis (orientation of the end effector)
end

== matlab function Four_DoF_02_2023b/MATLAB Function ==
  data: x input; joint_angles output; y input; z input; phi input
function joint_angles = IK_Simulink(x, y, z, phi)
    % IK_Simulink: Calculates joint angles for a 4-DOF manipulator
    
    % Lengths of the links
    L1 = 0.25; % Link 1
    L2 = 1; % Link 2
    L3 = 1.5; % Link 3
    L4 = 0.75; % Link 4 (End Effector)
    
    % 1. Calculate q1 (base rotation)
    q1 = atan2(y, x); % Base rotation angle
    
    % Project the target onto the xy-plane
    xe = sqrt(x^2 + y^2); % Projected target on the xy-plane
    ze = z - L1; % Remove L1 to focus on the target in the xy-plane

    % 2. Calculate the distance between joint 2 and the target (xe, ze)
    r = sqrt(xe^2 + ze^2);
    
    % Check if the target is within reach
    if r > (L2 + L3 + L4)
        error('Target position is out of reach.');
    end
    
    % 3. Use the Law of Cosines to calculate q3 (elbow joint)
    cos_theta3 = (r^2 - L2^2 - L3^2) / (2 * L2 * L3);
    q3 = atan2(-sqrt(1 - cos_theta3^2), cos_theta3); % Elbow-down configuration
    
    % 4. Calculate q2 (shoulder joint)
    beta = atan2(ze, xe); % Angle between the target and joint 2
    alpha = atan2(L3 * sin(q3), L2 + L3 * cos(q3)); % Angle from L2 to L3
    q2 = beta - alpha; % Final angle for joint 2
    
    % 5. Calculate q4 (end effector orientation)
    q4 = phi - (q2 + q3); % End effector rotation
    
    % Return joint angles as a vector
    joint_angles = [q1; q2; q3; q4];
end

== matlab function Four_DoF_02_2023b/MATLAB Function2 ==
  data: joint_angles input; FK output
function FK = FK_Simulink(joint_angles)
    mdl = "Four DoF 2";
    load_system(mdl);
    fk = simscape.multibody.KinematicsSolver(mdl);
    frameVariables(fk)
    jointPositionVariables(fk)
    FK = solve(fk,joint_angles);
end
